simulink model "polyinterp_1_"  (Simulink 7.8)
settings: Solver=ode45  StartTime=0.0  StopTime=2.0  RelTol=1e-3
values from neighbouring files (symbols this model uses):
  h = firpm(64,f,m)    [CFIR_1.m]    (also in adapt_filter1.m = adaptfilt.lms(ni,mu); adapt_filter2.m = adaptfilt.blms(ni,mu,1,36); adaptiv_2.m = [1 2 3 4 5 6 7 8 9 10]; adaptiv_3.m = [1 2 3 4 5 6 7 8 9 10])
  Ts = 1/fs    (= 6.25e-05)    [G722_1.m]    (also in adaptiv_2.m = 0.001; adaptiv_3.m = 0.001; adaptiv_4.m = 0.001; adaptiv_5.m = 0.001)
undefined symbols (not defined in the file or in its folder): g
libraries: dspsigops x7
settings Model: Creator=svenhoffmann  LastModifiedBy=josef  ExtModeAutoUpdateStatusClock=off
settings DataIOCC: SignalLoggingName=sigsOut
settings OptimizationCC: InitFltsAndDblsToZero=on
settings DebuggingCC: SaveWithParameterizedLinksMsg=none  SignalResolutionControl=TryResolveAllWithWarning  SolverPrmCheckMsg=none  MultiTaskDSMMsg=warning  MultiTaskCondExecSysMsg=none  FcnCallInpInsideContextMsg=Use local settings  StrictBusMsg=None
settings HardwareCC: TargetUnknown=on
settings RTWCC: IncludeERTFirstTime=on
settings GRTTargetCC: TargetFcnLib=ansi_tfl_tmw.mat

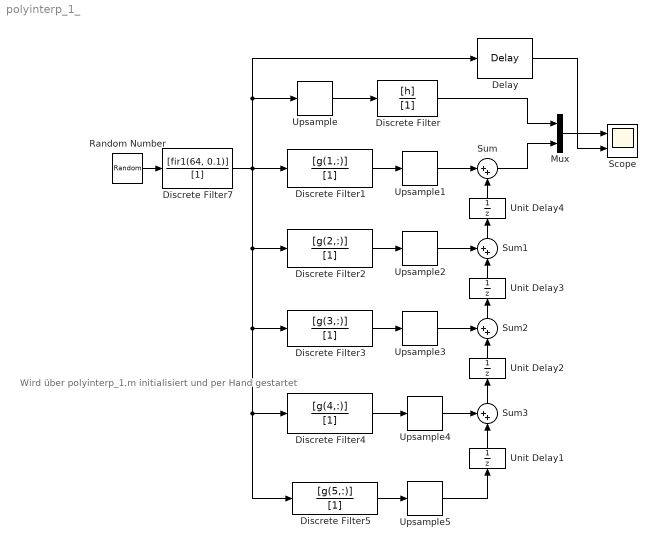
== system polyinterp_1_ ==
  note: Wird über polyinterp_1.m
      | initialisiert und per Hand gestartet
  Delay : dspsigops/Delay  InputProcessing=Inherited (this choice will be removed - see release notes)  dly_unit=Samples  delay=13  ic_detail=off  dif_ic_for_ch=off  dif_ic_for_dly=off  ic=0  reset_popup=None
  Discrete Filter : DiscreteFilter  Numerator=[h]  Denominator=[1]  SampleTime=Ts/5
  Discrete Filter1 : DiscreteFilter  Numerator=[g(1,:)]  Denominator=[1]  SampleTime=Ts
  Discrete Filter2 : DiscreteFilter  Numerator=[g(2,:)]  Denominator=[1]  SampleTime=Ts
  Discrete Filter3 : DiscreteFilter  Numerator=[g(3,:)]  Denominator=[1]  SampleTime=Ts
  Discrete Filter4 : DiscreteFilter  Numerator=[g(4,:)]  Denominator=[1]  SampleTime=Ts
  Discrete Filter5 : DiscreteFilter  Numerator=[g(5,:)]  Denominator=[1]  SampleTime=Ts
  Discrete Filter7 : DiscreteFilter  Numerator=[fir1(64, 0.1)]  Denominator=[1]  SampleTime=Ts
  Mux : Mux  Inputs=2
  Random Number : RandomNumber  SampleTime=Ts
  Scope : Scope  NumInputPorts=2
      settings: YMin=-0.2~-1  YMax=0.2~1
  Sum : Sum  Inputs=|++  SaturateOnIntegerOverflow=on
  Sum1 : Sum  Inputs=++|  SaturateOnIntegerOverflow=on
  Sum2 : Sum  Inputs=++|  SaturateOnIntegerOverflow=on
  Sum3 : Sum  Inputs=++|  SaturateOnIntegerOverflow=on
  Unit Delay{1..4} (4 alike) : UnitDelay  SampleTime=Ts/5
  Upsample{,1..5} (6 alike) : dspsigops/Upsample  N=5  phase=0  InputProcessing=Inherited (this choice will be removed - see release notes)  RateOptions=Allow multirate processing  ic=0  mode=Unused parameter value
  wires:
  Random Number/1 -> Discrete Filter7/1
  Discrete Filter/1 -> Mux/1
  Discrete Filter1/1 -> Upsample1/1
  Discrete Filter2/1 -> Upsample2/1
  Sum1/1 -> Unit Delay4/1
  Discrete Filter3/1 -> Upsample3/1
  Sum2/1 -> Unit Delay3/1
  Discrete Filter4/1 -> Upsample4/1
  Sum3/1 -> Unit Delay2/1
  Discrete Filter5/1 -> Upsample5/1
  Sum/1 -> Mux/2
  Mux/1 -> Scope/1
  Upsample/1 -> Discrete Filter/1
  Unit Delay4/1 -> Sum/2
  Unit Delay3/1 -> Sum1/2
  Unit Delay2/1 -> Sum2/2
  Unit Delay1/1 -> Sum3/2
  Upsample1/1 -> Sum/1
  Upsample2/1 -> Sum1/1
  Upsample3/1 -> Sum2/1
  Upsample4/1 -> Sum3/1
  Upsample5/1 -> Unit Delay1/1
  Discrete Filter7/1 -> Discrete Filter1/1, Upsample/1, Delay/1, Discrete Filter2/1, Discrete Filter3/1, Discrete Filter4/1, Discrete Filter5/1
  Delay/1 -> Scope/2
